simulink model "behavior_IMM_Pred_HighD"  (R2019b)
settings: Solver=FixedStepAuto  StartTime=0.0  StopTime=10  FixedStep=Ts_bp  RelTol=1e-3
undefined symbols (not defined in the file or in its folder): P_init, sigbuilder_block, Ts_bp, vx, vy, x, y
libraries: simulink x2
settings Model: Creator=jasprit  LastModifiedBy=jasprit

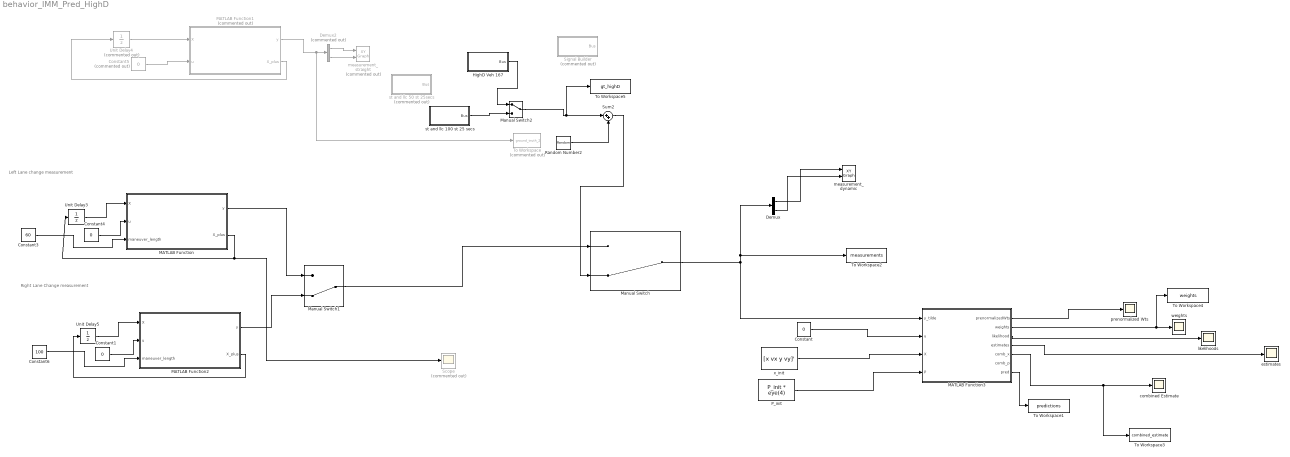
== system behavior_IMM_Pred_HighD ==
  note: Left Lane change measurement
  note: Right Lane Change measurement
  Constant : Constant  Value=0
  Constant1 : Constant  Value=0  SampleTime=-1
  Constant3 : Constant  Value=60  SampleTime=-1
  Constant4 : Constant  Value=0  SampleTime=-1
  Constant5 : Constant  Commented=on  Value=0  SampleTime=-1
  Constant6 : Constant  Value=100  SampleTime=-1
  Demux : Demux  Outputs=2
  Demux2 : Demux  Commented=on  Outputs=2
  HighD Veh 167 : Subsystem  Tag=STV Subsys  LoadFcn=sigbuilder_block('load');  StartFcn=sigbuilder_block('start');  StopFcn=sigbuilder_block('stop');  ClipboardFcn=sigbuilder_block('clipboard');  mask(Sigbuilder block){tuvar=[0:10]}
      mask help: Simulink:masks:SigbuilderBlock_MD
      mask init:
      | if ~strcmp(get_param(bdroot(gcbh),'SimulationStatus'),'stopped') tuvar = sigbuilder_block('maskInit'); end
      settings: CopyFcn=sigbuilder_block('copy');  DeleteFcn=sigbuilder_block('delete');  ModelCloseFcn=sigbuilder_block('modelClose');  PreSaveFcn=sigbuilder_block('preSave');  PauseFcn=sigbuilder_block('pause');  ContinueFcn=sigbuilder_block('continue');  NameChangeFcn=sigbuilder_block('namechange');  OpenFcn=sigbuilder_block('open',[67.5 0 588 512.25 ]);  CloseFcn=sigbuilder_block('close');
      mask Display: plot(0, 0, 100, 100,[2, 2, 32, 32, 2], [68, 8, 8, 68, 68],[32, 2], [38, 38], [32, 19, 2],[53, 60, 44], [32, 17, 17, 2],[16, 16, 31, 31]);txt = getActiveGroup(gcbh);text(2, 100, txt,'verticalAlignment', 'top');
  MATLAB Function : MATLAB Function  TreatAsAtomicUnit=on
  MATLAB Function1 : MATLAB Function  Commented=on  TreatAsAtomicUnit=on
  MATLAB Function2 : MATLAB Function  TreatAsAtomicUnit=on
  MATLAB Function3 : MATLAB Function  TreatAsAtomicUnit=on
  Manual Switch : ManualSwitch  CurrentSetting=0
  Manual Switch1 : ManualSwitch  CurrentSetting=0
  Manual Switch2 : ManualSwitch
  P_init : Constant  Value=P_init * eye(4)  SampleTime=-1
  Random Number2 : RandomNumber  Variance=0.0025  SampleTime=Ts_bp
  Scope : Scope  Commented=on
  Signal Builder : Subsystem  Tag=STV Subsys  Commented=on  LoadFcn=sigbuilder_block('load');  StartFcn=sigbuilder_block('start');  StopFcn=sigbuilder_block('stop');  ClipboardFcn=sigbuilder_block('clipboard');  mask(Sigbuilder block){tuvar=[0:10]}
      mask help: Simulink:masks:SigbuilderBlock_MD
      mask init:
      | if ~strcmp(get_param(bdroot(gcbh),'SimulationStatus'),'stopped') tuvar = sigbuilder_block('maskInit'); end
      settings: CopyFcn=sigbuilder_block('copy');  DeleteFcn=sigbuilder_block('delete');  ModelCloseFcn=sigbuilder_block('modelClose');  PreSaveFcn=sigbuilder_block('preSave');  PauseFcn=sigbuilder_block('pause');  ContinueFcn=sigbuilder_block('continue');  NameChangeFcn=sigbuilder_block('namechange');  OpenFcn=sigbuilder_block('open',[411 7.5 573 467.25 ]);  CloseFcn=sigbuilder_block('close');
      mask Display: plot(0, 0, 100, 100,[2, 2, 32, 32, 2], [68, 8, 8, 68, 68],[32, 2], [38, 38], [32, 19, 2],[53, 60, 44], [32, 17, 17, 2],[16, 16, 31, 31]);txt = getActiveGroup(gcbh);text(2, 100, txt,'verticalAlignment', 'top');
  Sum2 : Sum  Inputs=|++
  To Workspace : ToWorkspace  Commented=on  VariableName=ground_truth_2  SaveFormat=Timeseries  SampleTime=-1
  To Workspace1 : ToWorkspace  VariableName=predictions  SaveFormat=Timeseries  SampleTime=-1
  To Workspace2 : ToWorkspace  VariableName=measurements  SaveFormat=Timeseries  SampleTime=-1
  To Workspace3 : ToWorkspace  VariableName=combined_estimate  SaveFormat=Timeseries  SampleTime=-1
  To Workspace4 : ToWorkspace  VariableName=weights  SaveFormat=Timeseries  SampleTime=-1
  To Workspace5 : ToWorkspace  VariableName=gt_highD  SaveFormat=Timeseries  SampleTime=-1
  Unit Delay3 : UnitDelay  InitialCondition=[x vx y vy]  SampleTime=Ts_bp  HasFrameUpgradeWarning=on
  Unit Delay4 : UnitDelay  Commented=on  InitialCondition=[x vx y vy]  SampleTime=-1  HasFrameUpgradeWarning=on
  Unit Delay5 : UnitDelay  InitialCondition=[x vx y vy]  SampleTime=Ts_bp  HasFrameUpgradeWarning=on
  combined Estimate : Scope
  estimates : Scope
  likelihoods : Scope
  measurement_dynamic : simulink/Sinks/XY Graph  xmin=-1  xmax=200  ymin=-5  ymax=5  st=-1
  measurement_straight : simulink/Sinks/XY Graph  Commented=on  xmin=-1  xmax=200  ymin=-5  ymax=5  st=-1
  prenormalized Wts : Scope
  st and llc 100 st 25 secs : Subsystem  Tag=STV Subsys  LoadFcn=sigbuilder_block('load');  StartFcn=sigbuilder_block('start');  StopFcn=sigbuilder_block('stop');  ClipboardFcn=sigbuilder_block('clipboard');  mask(Sigbuilder block){tuvar=[0:10]}
      mask help: Simulink:masks:SigbuilderBlock_MD
      mask init:
      | if ~strcmp(get_param(bdroot(gcbh),'SimulationStatus'),'stopped') tuvar = sigbuilder_block('maskInit'); end
      settings: CopyFcn=sigbuilder_block('copy');  DeleteFcn=sigbuilder_block('delete');  ModelCloseFcn=sigbuilder_block('modelClose');  PreSaveFcn=sigbuilder_block('preSave');  PauseFcn=sigbuilder_block('pause');  ContinueFcn=sigbuilder_block('continue');  NameChangeFcn=sigbuilder_block('namechange');  OpenFcn=sigbuilder_block('open',[437.25 157.5 550.5 399.75 ]);  CloseFcn=sigbuilder_block('close');
      mask Display: plot(0, 0, 100, 100,[2, 2, 32, 32, 2], [68, 8, 8, 68, 68],[32, 2], [38, 38], [32, 19, 2],[53, 60, 44], [32, 17, 17, 2],[16, 16, 31, 31]);txt = getActiveGroup(gcbh);text(2, 100, txt,'verticalAlignment', 'top');
  st and llc 50 st 25secs : Subsystem  Tag=STV Subsys  Commented=on  LoadFcn=sigbuilder_block('load');  StartFcn=sigbuilder_block('start');  StopFcn=sigbuilder_block('stop');  ClipboardFcn=sigbuilder_block('clipboard');  mask(Sigbuilder block){tuvar=[0:10]}
      mask help: Simulink:masks:SigbuilderBlock_MD
      mask init:
      | if ~strcmp(get_param(bdroot(gcbh),'SimulationStatus'),'stopped') tuvar = sigbuilder_block('maskInit'); end
      settings: CopyFcn=sigbuilder_block('copy');  DeleteFcn=sigbuilder_block('delete');  ModelCloseFcn=sigbuilder_block('modelClose');  PreSaveFcn=sigbuilder_block('preSave');  PauseFcn=sigbuilder_block('pause');  ContinueFcn=sigbuilder_block('continue');  NameChangeFcn=sigbuilder_block('namechange');  OpenFcn=sigbuilder_block('open',[433.5 132.75 558 422.25 ]);  CloseFcn=sigbuilder_block('close');
      mask Display: plot(0, 0, 100, 100,[2, 2, 32, 32, 2], [68, 8, 8, 68, 68],[32, 2], [38, 38], [32, 19, 2],[53, 60, 44], [32, 17, 17, 2],[16, 16, 31, 31]);txt = getActiveGroup(gcbh);text(2, 100, txt,'verticalAlignment', 'top');
  weights : Scope
  x_init : Constant  Value=[x vx y vy]'
  wires:
  Unit Delay3/1 -> MATLAB Function/1(X)
  MATLAB Function2/1(y) -> Manual Switch1/2
  Demux2/1 -> measurement_straight/1
  Constant/1 -> MATLAB Function3/2(u)
  Unit Delay5/1 -> MATLAB Function2/1(X)
  MATLAB Function1/1(y) -> To Workspace/1, Demux2/1
  Constant1/1 -> MATLAB Function2/2(u)
  Constant6/1 -> MATLAB Function2/3(maneuver_length)
  MATLAB Function/1(y) -> Manual Switch1/1
  Manual Switch/1 -> MATLAB Function3/1(y_tilde), Demux/1, To Workspace2/1
  Constant4/1 -> MATLAB Function/2(u)
  Unit Delay4/1 -> MATLAB Function1/1(X)
  Demux/1 -> measurement_dynamic/1
  Constant3/1 -> MATLAB Function/3(maneuver_length)
  MATLAB Function1/2(X_plus) -> Unit Delay4/1
  MATLAB Function/2(X_plus) -> Scope/1, Unit Delay3/1
  Sum2/1 -> Manual Switch/2
  Random Number2/1 -> Sum2/2
  Constant5/1 -> MATLAB Function1/2(u)
  MATLAB Function2/2(X_plus) -> Unit Delay5/1
  Demux2/2 -> measurement_straight/2
  Demux/2 -> measurement_dynamic/2
  Manual Switch1/1 -> Manual Switch/1
  P_init/1 -> MATLAB Function3/4(P)
  MATLAB Function3/1(prenormalizedWts) -> prenormalized Wts/1
  MATLAB Function3/2(weights) -> To Workspace4/1, weights/1
  MATLAB Function3/3(likelihood) -> likelihoods/1
  MATLAB Function3/4(estimates) -> estimates/1
  x_init/1 -> MATLAB Function3/3(X)
  MATLAB Function3/5(comb_x) -> To Workspace3/1, combined Estimate/1
  st and llc 100 st 25 secs/1(Bus) -> Manual Switch2/2
  Manual Switch2/1 -> To Workspace5/1, Sum2/1
  MATLAB Function3/7(pred) -> To Workspace1/1
  HighD Veh 167/1(Bus) -> Manual Switch2/1

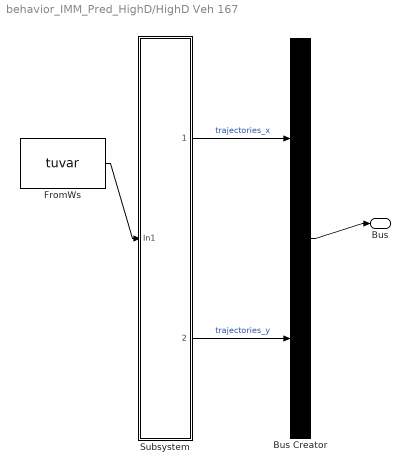
== system behavior_IMM_Pred_HighD/HighD Veh 167 ==
  Bus Creator : BusCreator  Tag=Bus Creator  Inputs=2
  FromWs : FromWorkspace  Tag=STV FromWs  VariableName=tuvar  SampleTime=0
      SigBuilderData=|
      | common.afterFinalStr = 'Extrapolate'
      | common.sampleTime = 0
      | dataSet.timeRange = [0 15]
      | dataSet.name = 'Group 1'
      | sbobj.Groups.Name = 'Group 1'
      | sbobj.Groups.Signals(1).Name = 'trajectories_x'
      | sbobj.Groups.Signals(1).XData = [0 0.04 0.08 0.12 0.16 0.2 0.24 0.28 0.32 0.36 0.4 0.44 0.48 0.52 0.56 0.6 0.64 0.68 0.72 0.76 0.8 0.84 0.88 0.92 0.96 1 1.04 1.08 1.12 1.16 1.2 1.24 1.28 1.32 1.36 1.4 1.44 1.48 1.52 1.56 1.6 1.64 1.68 1.72 1.76 1.8 1.84 1.88 1.92 1.96 2 2.04 2.08 2.12 2.16 2.2 2.24 2.28 2.32 2.36 2.4 2.44 2.48 2.52 2.56 2.6 2.64 2.68 2.72 2.76 2.8 2.84 2.88 2.92 2.96 3 3.04 3.08 3.12 3.16 3.2 3.24 3.28 3.32 3.36 3.4 3.44 3.48 3.52 3.56 3.6 3.64 3.68 3.72 3.76 3.8 3.84 3.88 3.92 3.96 4 4.04 4.08 4.12 4.16 4.2 4.24 4.28 4.32 4.36 4.4 4.44 4.48 4.52 4.56 4.6 4.64 4.68 4.72 4.76 4.8 4.84 4.88 4.92 4.96 5 5.04 5.08 5.12 5.16 5.2 5.24 5.28 5.32 5.36 5.4 5.44 5.48 5.52 5.56 5.6 5.64 5.68 5.72 5.76 5.8 5.84 5.88 5.92 5.96 6 6.04 6.08 6.12 6.16 6.2 6.24 6.28 6.32 6.36 6.4 6.44 6.48 6.52 6.56 6.6 6.64 6.68 6.72 6.76 6.8 6.84 6.88 6.92 6.96 7 7.04 7.08 7.12 7.16 7.2 7.24 7.28 7.32 7.36 7.4 7.44 7.48 7.52 7.56 7.6 7.64 7.68 7.72 7.76 7.8 7.84 7.88 7.92 7.96 8 8.04 8.08 8.12 8.16 8.2 8.24 8.28 8.32 8.36 8.4 8.44 8.48 8.52 8.56 8.6 8.64 8.68 8.72 8.76 8.8 8.84 8.88 8.92 8.96 9 9.04 9.08 9.12 9.16 9.2 9.24 9.28 9.32 9.36 9.4 9.44 9.48 9.52 9.56 9.6 9.64 9.68 9.72 9.76 9.8 9.84 9.88 9.92 9.96 10 10.04 10.08 10.12 10.16 10.2 10.24 10.28 15]
      | sbobj.Groups.Signals(1).YData = [6.005 7.345 8.725 10.135 11.565 12.995 14.425 15.875 17.325 18.795 20.245 21.715 ... (259 elements, 1x259)]
      | sbobj.Groups.Signals(2).Name = 'trajectories_y'
      | sbobj.Groups.Signals(2).XData = [0 0.04 0.08 0.12 0.16 0.2 0.24 0.28 0.32 0.36 0.4 0.44 0.48 0.52 0.56 0.6 0.64 0.68 0.72 0.76 0.8 0.84 0.88 0.92 0.96 1 1.04 1.08 1.12 1.16 1.2 1.24 1.28 1.32 1.36 1.4 1.44 1.48 1.52 1.56 1.6 1.64 1.68 1.72 1.76 1.8 1.84 1.88 1.92 1.96 2 2.04 2.08 2.12 2.16 2.2 2.24 2.28 2.32 2.36 2.4 2.44 2.48 2.52 2.56 2.6 2.64 2.68 2.72 2.76 2.8 2.84 2.88 2.92 2.96 3 3.04 3.08 3.12 3.16 3.2 3.24 3.28 3.32 3.36 3.4 3.44 3.48 3.52 3.56 3.6 3.64 3.68 3.72 3.76 3.8 3.84 3.88 3.92 3.96 4 4.04 4.08 4.12 4.16 4.2 4.24 4.28 4.32 4.36 4.4 4.44 4.48 4.52 4.56 4.6 4.64 4.68 4.72 4.76 4.8 4.84 4.88 4.92 4.96 5 5.04 5.08 5.12 5.16 5.2 5.24 5.28 5.32 5.36 5.4 5.44 5.48 5.52 5.56 5.6 5.64 5.68 5.72 5.76 5.8 5.84 5.88 5.92 5.96 6 6.04 6.08 6.12 6.16 6.2 6.24 6.28 6.32 6.36 6.4 6.44 6.48 6.52 6.56 6.6 6.64 6.68 6.72 6.76 6.8 6.84 6.88 6.92 6.96 7 7.04 7.08 7.12 7.16 7.2 7.24 7.28 7.32 7.36 7.4 7.44 7.48 7.52 7.56 7.6 7.64 7.68 7.72 7.76 7.8 7.84 7.88 7.92 7.96 8 8.04 8.08 8.12 8.16 8.2 8.24 8.28 8.32 8.36 8.4 8.44 8.48 8.52 8.56 8.6 8.64 8.68 8.72 8.76 8.8 8.84 8.88 8.92 8.96 9 9.04 9.08 9.12 9.16 9.2 9.24 9.28 9.32 9.36 9.4 9.44 9.48 9.52 9.56 9.6 9.64 9.68 9.72 9.76 9.8 9.84 9.88 9.92 9.96 10 10.04 10.08 10.12 10.16 10.2 10.24 15]
      | sbobj.Groups.Signals(2).YData = [22.64 22.64 22.64 22.64 22.64 22.64 22.64 22.64 22.65 22.65 22.65 22.65 22.65 22.65 22.66 22.66 22.66 22.67 22.67 22.68 22.68 22.69 22.69 22.7 22.7 22.71 22.71 22.72 22.73 22.74 22.74 22.75 22.76 22.77 22.78 22.79 22.8 22.81 22.82 22.83 22.84 22.85 22.86 22.87 22.89 22.9 22.91 22.92 22.94 22.95 22.96 22.98 22.99 23.01 23.02 23.04 23.05 23.07 23.08 23.1 23.12 23.14 23.15 23.17 23.19 23.21 23.24 23.26 23.28 23.3 23.33 23.35 23.38 23.4 23.43 23.46 23.49 23.51 23.54 23.57 23.6 23.63 23.67 23.7 23.73 23.76 23.79 23.83 23.86 23.9 23.93 23.97 24 24.04 24.07 24.11 24.15 24.18 24.22 24.26 24.29 24.33 24.37 24.41 24.44 24.48 24.52 24.56 24.59 24.63 24.67 24.71 24.74 24.78 24.82 24.86 24.9 24.93 24.97 25.01 25.05 25.09 25.12 25.16 25.2 25.24 25.27 25.31 25.34 25.38 25.41 25.44 25.48 25.51 25.54 25.57 25.6 25.63 25.66 25.69 25.72 25.74 25.77 25.8 25.82 25.85 25.87 25.9 25.92 25.94 25.96 25.99 26.01 26.03 26.05 26.07 26.09 26.11 26.12 26.14 26.16 26.17 26.19 26.2 26.22 26.23 26.24 26.25 26.26 26.27 26.28 26.29 26.3 26.31 26.32 26.33 26.34 26.34 26.35 26.36 26.36 26.37 26.37 26.38 26.38 26.39 26.39 26.4 26.4 26.41 26.41 26.41 26.42 26.42 26.42 26.42 26.43 26.43 26.43 26.43 26.43 26.44 26.44 26.44 26.44 26.44 26.44 26.45 26.45 26.45 26.45 26.45 26.45 26.45 26.45 26.46 26.46 26.46 26.46 26.46 26.46 26.47 26.47 26.47 26.47 26.47 26.47 26.47 26.48 26.48 26.48 26.48 26.48 26.48 26.48 26.48 26.48 26.48 26.48 26.48 26.48 26.48 26.48 26.48 26.48 26.48 26.48 26.48 26.48 26.48 26.48 26.48 26.48 26.47 26.47 26.47 26.47 26.47]
      | sbobj.Groups.TimeRange = [0 15]
  Subsystem : Subsystem
  Bus : Outport
  wires:
  FromWs/1 -> Subsystem/1(In1)
  Subsystem/1(trajectories_x) -> Bus Creator/1  "trajectories_x"
  Subsystem/2(trajectories_y) -> Bus Creator/2  "trajectories_y"
  Bus Creator/1 -> Bus/1

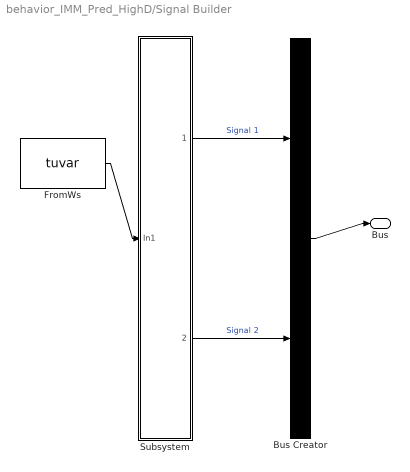
== system behavior_IMM_Pred_HighD/Signal Builder ==
  Bus Creator : BusCreator  Tag=Bus Creator  Inputs=2
  FromWs : FromWorkspace  Tag=STV FromWs  VariableName=tuvar  SampleTime=0
      SigBuilderData=|
      | common.afterFinalStr = 'Extrapolate'
      | common.sampleTime = 0
      | dataSet.timeRange = [0 20]
      | dataSet.name = 'Group 1'
      | sbobj.Groups.Name = 'Group 1'
      | sbobj.Groups.Signals(1).Name = 'Signal 1'
      | sbobj.Groups.Signals(1).XData = [0 0.01 0.02 0.03 0.04 0.05 0.06 0.07 0.08 0.09 0.1 0.11 ... (2001 elements, 1x2001)]
      | sbobj.Groups.Signals(1).YData = [0 0.1 0.2 0.3 0.4 0.5 0.6 0.7 0.8 0.9 1 1.1 ... (2001 elements, 1x2001)]
      | sbobj.Groups.Signals(2).Name = 'Signal 2'
      | sbobj.Groups.Signals(2).XData = [0 0.01 0.02 0.03 0.04 0.05 0.06 0.07 0.08 0.09 0.1 0.11 ... (2001 elements, 1x2001)]
      | sbobj.Groups.Signals(2).YData = [0 0 0 0 0 0 0 0 0 0 0 0 ... (2001 elements, 1x2001)]
      | sbobj.Groups.TimeRange = [0 20]
  Subsystem : Subsystem
  Bus : Outport  VectorParamsAs1DForOutWhenUnconnected=off
  wires:
  FromWs/1 -> Subsystem/1(In1)
  Bus Creator/1 -> Bus/1
  Subsystem/1(Signal 1) -> Bus Creator/1  "Signal 1"
  Subsystem/2(Signal 2) -> Bus Creator/2  "Signal 2"

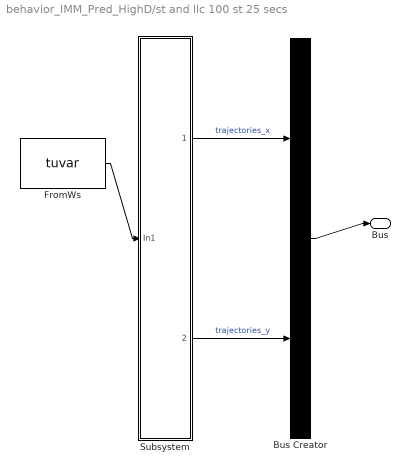
== system behavior_IMM_Pred_HighD/st and llc 100 st 25 secs ==
  Bus Creator : BusCreator  Tag=Bus Creator  Inputs=2
  FromWs : FromWorkspace  Tag=STV FromWs  VariableName=tuvar  SampleTime=0
      SigBuilderData=|
      | common.afterFinalStr = 'Extrapolate'
      | common.sampleTime = 0
      | dataSet.timeRange = [0 25]
      | dataSet.name = 'Group 1'
      | sbobj.Groups.Name = 'Group 1'
      | sbobj.Groups.Signals(1).Name = 'trajectories_x'
      | sbobj.Groups.Signals(1).XData = [0 0.01 0.02 0.03 0.04 0.05 0.06 0.07 0.08 0.09 0.1 0.11 ... (2501 elements, 1x2501)]
      | sbobj.Groups.Signals(1).YData = [0 0.1 0.2 0.3 0.4 0.5 0.6 0.7 0.8 0.9 1 1.1 ... (2501 elements, 1x2501)]
      | sbobj.Groups.Signals(2).Name = 'trajectories_y'
      | sbobj.Groups.Signals(2).XData = [0 0.01 0.02 0.03 0.04 0.05 0.06 0.07 0.08 0.09 0.1 0.11 ... (2501 elements, 1x2501)]
      | sbobj.Groups.Signals(2).YData = [0 0 0 0 0 0 0 0 0 0 0 0 ... (2501 elements, 1x2501)]
      | sbobj.Groups.TimeRange = [0 25]
  Subsystem : Subsystem
  Bus : Outport
  wires:
  FromWs/1 -> Subsystem/1(In1)
  Subsystem/1(trajectories_x) -> Bus Creator/1  "trajectories_x"
  Subsystem/2(trajectories_y) -> Bus Creator/2  "trajectories_y"
  Bus Creator/1 -> Bus/1

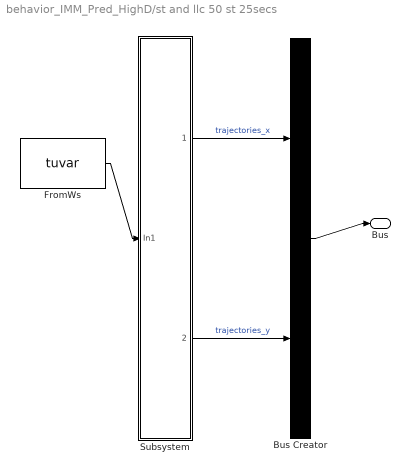
== system behavior_IMM_Pred_HighD/st and llc 50 st 25secs ==
  Bus Creator : BusCreator  Tag=Bus Creator  Inputs=2
  FromWs : FromWorkspace  Tag=STV FromWs  VariableName=tuvar  SampleTime=0
      SigBuilderData=|
      | common.afterFinalStr = 'Extrapolate'
      | common.sampleTime = 0
      | dataSet.timeRange = [0 25]
      | dataSet.name = 'Group 1'
      | sbobj.Groups.Name = 'Group 1'
      | sbobj.Groups.Signals(1).Name = 'trajectories_x'
      | sbobj.Groups.Signals(1).XData = [0 0.01 0.02 0.03 0.04 0.05 0.06 0.07 0.08 0.09 0.1 0.11 ... (2501 elements, 1x2501)]
      | sbobj.Groups.Signals(1).YData = [0 0.1 0.2 0.3 0.4 0.5 0.6 0.7 0.8 0.9 1 1.1 ... (2501 elements, 1x2501)]
      | sbobj.Groups.Signals(2).Name = 'trajectories_y'
      | sbobj.Groups.Signals(2).XData = [0 0.01 0.02 0.03 0.04 0.05 0.06 0.07 0.08 0.09 0.1 0.11 ... (2501 elements, 1x2501)]
      | sbobj.Groups.Signals(2).YData = [0 0 0 0 0 0 0 0 0 0 0 0 ... (2501 elements, 1x2501)]
      | sbobj.Groups.TimeRange = [0 25]
  Subsystem : Subsystem
  Bus : Outport
  wires:
  FromWs/1 -> Subsystem/1(In1)
  Subsystem/1(trajectories_x) -> Bus Creator/1  "trajectories_x"
  Subsystem/2(trajectories_y) -> Bus Creator/2  "trajectories_y"
  Bus Creator/1 -> Bus/1

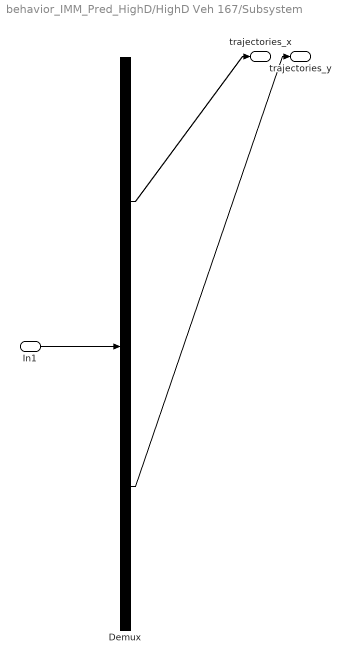
== system behavior_IMM_Pred_HighD/HighD Veh 167/Subsystem ==
  In1 : Inport
  Demux : Demux  Tag=STV Demux  Outputs=2
  trajectories_x : Outport  Tag=STV Outport
  trajectories_y : Outport  Tag=STV Outport  Port=2
  wires:
  Demux/1 -> trajectories_x/1
  Demux/2 -> trajectories_y/1
  In1/1 -> Demux/1

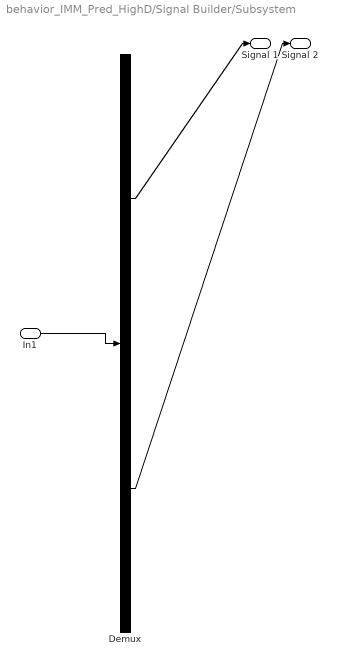
== system behavior_IMM_Pred_HighD/Signal Builder/Subsystem ==
  In1 : Inport
  Demux : Demux  Tag=STV Demux  Outputs=2
  Signal 1 : Outport  Tag=STV Outport  VectorParamsAs1DForOutWhenUnconnected=off
  Signal 2 : Outport  Tag=STV Outport  Port=2  VectorParamsAs1DForOutWhenUnconnected=off
  wires:
  In1/1 -> Demux/1
  Demux/1 -> Signal 1/1
  Demux/2 -> Signal 2/1

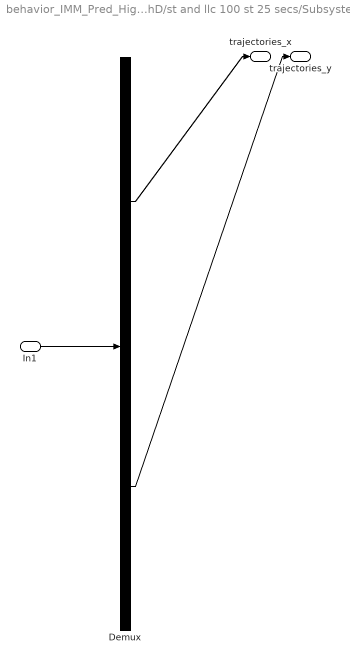
== system behavior_IMM_Pred_HighD/st and llc 100 st 25 secs/Subsystem ==
  In1 : Inport
  Demux : Demux  Tag=STV Demux  Outputs=2
  trajectories_x : Outport  Tag=STV Outport
  trajectories_y : Outport  Tag=STV Outport  Port=2
  wires:
  Demux/1 -> trajectories_x/1
  Demux/2 -> trajectories_y/1
  In1/1 -> Demux/1

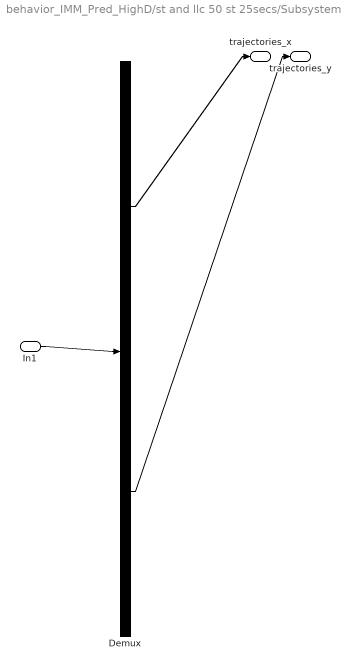
== system behavior_IMM_Pred_HighD/st and llc 50 st 25secs/Subsystem ==
  In1 : Inport
  Demux : Demux  Tag=STV Demux  Outputs=2
  trajectories_x : Outport  Tag=STV Outport
  trajectories_y : Outport  Tag=STV Outport  Port=2
  wires:
  Demux/1 -> trajectories_x/1
  Demux/2 -> trajectories_y/1
  In1/1 -> Demux/1

== matlab function behavior_IMM_Pred_HighD/MATLAB Function ==
  data: X input; u input; y output; X_plus output; maneuver_length input
function [y, X_plus]= measurementsForLaneChange(X, u, maneuver_length)

    Ts_bp = 0.1;
%     maneuver_length = 150;  %m
    lane_center_to_center_distance = 3.5;   %meters

    % states - X = [x vx y vy] -     
    Ck = [1 0 0 0; 0 0 1 0];

    % measurement noise std_dev
%     R_sigma = [0.5 0; 0 0.5];
   R_sigma = [0.05 0; 0 0.05];
    
    % process noise std dev
%    sigma_matrix = diag([0.16 0.16 0.16 0.16]);
    sigma_matrix = diag([0.032 0.032 0.032 0.032]);
    
%     if t < 15
%         Ak = [1 Ts 0 0; 0 1 0 0; 0 0 1 Ts; 0 0 0 1];
%         Bk = 0;
%         X_plus = Ak * X + Bk * u + sqrt(Ts) * sigma_matrix * randn(4,1);
%     else
        X_plus = leftLaneChangeParametricFcn(X, u, maneuver_length, lane_center_to_center_distance) + sqrt(Ts_bp)*sigma_matrix*randn(4,1);    
%     end
    
    y = Ck * X_plus + R_sigma * randn(2,1);
    
end

== matlab function behavior_IMM_Pred_HighD/MATLAB Function1 ==
  data: X input; u input; y output; X_plus output
function [y, X_plus]= measurementsForStraightMotion(X, u)

    Ts_bp = 0.1;
    % states - X = [x vx y vy] -     
    Ak = [1 Ts_bp 0 0; 0 1 0 0; 0 0 1 Ts_bp; 0 0 0 1];
    Bk = 0;
    Ck = [1 0 0 0; 0 0 1 0];

    % measurement noise std_dev
%     R_sigma = [0.5 0; 0 0.5];
   R_sigma = [0.05 0; 0 0.05];
    
    % process noise std dev
%    sigma_matrix = diag([0.16 0.16 0.16 0.16]);
    sigma_matrix = diag([0.032 0.032 0.032 0.032]);
  
    X(3) = 0;
%    X(4) = 0;
    
    X_plus = Ak * X + Bk * u + sqrt(Ts_bp)*sigma_matrix*randn(4,1);    
    
    y = Ck * X_plus + R_sigma * randn(2,1);
    
end

== matlab function behavior_IMM_Pred_HighD/MATLAB Function2 ==
  data: X input; u input; y output; X_plus output; maneuver_length input
function [y, X_plus]= measurementsForLaneChange(X, u, maneuver_length)

    Ts_bp = 0.1;
%    maneuver_length = 150;  %m
    lane_center_to_center_distance = 3.5;   %meters

    % states - X = [x vx y vy] -     
    Ck = [1 0 0 0; 0 0 1 0];

    % measurement noise std_dev
%     R_sigma = [0.5 0; 0 0.5];
   R_sigma = [0.05 0; 0 0.05];
    
    % process noise std dev
%    sigma_matrix = diag([0.16 0.16 0.16 0.16]);
    sigma_matrix = diag([0.032 0.032 0.032 0.032]);
    
%     if t < 15
%         Ak = [1 Ts 0 0; 0 1 0 0; 0 0 1 Ts; 0 0 0 1];
%         Bk = 0;
%         X_plus = Ak * X + Bk * u + sqrt(Ts) * sigma_matrix * randn(4,1);
%     else
        X_plus = rightLaneChangeParametricFcn(X, u, maneuver_length, lane_center_to_center_distance) + sqrt(Ts_bp)*sigma_matrix*randn(4,1);    
%     end
    
    y = Ck * X_plus + R_sigma * randn(2,1);
    
end

== matlab function behavior_IMM_Pred_HighD/MATLAB Function3 ==
  data: y_tilde input; u input; prenormalizedWts output; X input; P input; weights output; likelihood output; estimates output; comb_x output; comb_p output; pred output
function [prenormalizedWts, weights, likelihood, estimates, comb_x, comb_p, pred]   = imm_laneChanges(y_tilde, u, X, P)
    persistent amm;
    
    if isempty(amm)
        Ts = 1/25;
        
        amm = HighDAllBehaviorsIMMPred(Ts);
    end
    
    
    pred = zeros(5, 125, 5);

    % mix initial states for the current cycle first
    amm.mixEstimates();

    % predict
    amm.predict(u);
    
    % correct and update probabilistic weights
    amm.correct(y_tilde);
    
    % combined estimates
    [comb_x, comb_p] = amm.calculateCombinedEstimate();
    
    prenormalizedWts = amm.getFilterNonNormalizedWeights();
    weights = amm.getFilterWeights();
    likelihood = amm.getFilterLikelihoods();
    estimates = amm.getFilterEstimates();
    pred = amm.getPredictions();
end
